simulink model "DIL_2025a"  (R2025a)
settings: Solver=VariableStepAuto  StartTime=0.0  StopTime=inf  FixedStep=.01  RelTol=1e-2
values from neighbouring files (symbols this model uses):
  s0 = load("s0.mat").s1(1:22)    [DIL_matlab.m]    (also in setup.m = load("s0.mat").s1(1:18)')
libraries: sl3dlib x1, sim3dlib x1, sim3dautolib x1
settings Model: Creator=Inver  LastModifiedBy=TAK
settings SolverCC: SolverJacobianMethodControl=FullAnalytical  DaesscMode=Robust  ZeroCrossAlgorithm=Adaptive
settings RTWCC: GPUComputeCapability=3.5

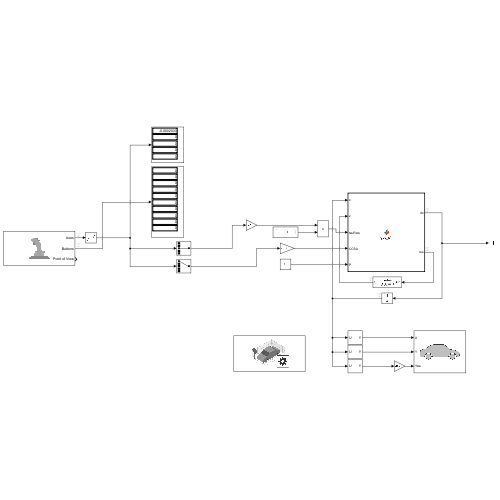
[thumbnail: Simulink's stored preview of the top-level diagram]
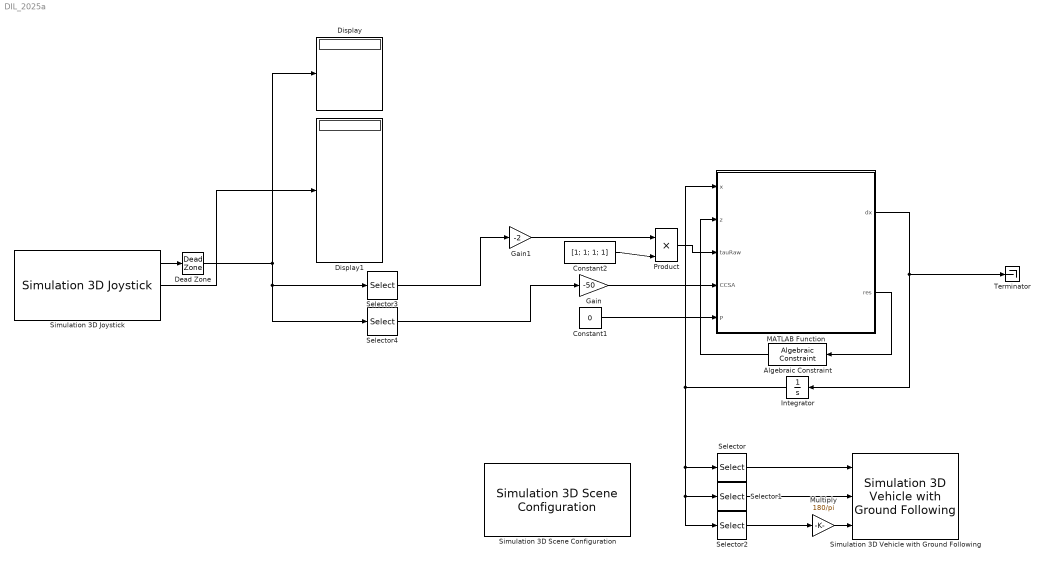
== system DIL_2025a ==
  Algebraic Constraint : AlgebraicConstraint  Tolerance=1e-6  InitialGuess=zeros(4, 1)
  Constant1 : Constant  Value=0
  Constant2 : Constant  Value=[1; 1; 1; 1]
  Dead Zone : DeadZone  LowerValue=-.02  UpperValue=.02
  Display : Display
  Display1 : Display
  Gain : Gain  Gain=-50
  Gain1 : Gain  Gain=-2
  Integrator : Integrator  InitialCondition=s0(1:18)
  MATLAB Function : MATLAB Function  TreatAsAtomicUnit=on
  Multiply : Gain  Gain=180/pi
  Product : Product
  Selector : Selector  InputPortWidth=18  IndexOptions=Index vector (dialog)  Indices=2  OutputSizes=1
  Selector1 : Selector  InputPortWidth=18  IndexOptions=Index vector (dialog)  Indices=4  OutputSizes=1
  Selector2 : Selector  InputPortWidth=18  IndexOptions=Index vector (dialog)  Indices=12  OutputSizes=1
  Selector3 : Selector  InputPortWidth=5  IndexOptions=Index vector (dialog)  Indices=3  OutputSizes=1
  Selector4 : Selector  InputPortWidth=5  IndexOptions=Index vector (dialog)  Indices=1  OutputSizes=1
  Simulation 3D Joystick : sl3dlib/Simulation 3D/Hardware Interface/Simulation 3D Joystick  joyid=1  adjustports=on  forcefeed=off
  Simulation 3D Scene Configuration : sim3dlib/Simulation 3D Scene Configuration  Priority=0  ProjectFormat=Default Scenes  SceneDesc=Double lane change  ProjectName=C:\Program Files\MATLAB\R2025a\toolbox\shared\sim3d_projects\automotive_project_windows\UE\WindowsNoEditor\VehicleSimulation.exe  ScenePath=/Game/Maps/HwStrght  EnableOpenDRIVE=off  vehTagList={'Custom';'Scene Origin';'SimulinkVehicle1'}  vehTag=SimulinkVehicle1  AttachedCameraRelativeTranslation=[0 0 10]  FreeCameraDefaultInitialTranslation=[-6, 0, 2]  AttachedCameraRelativeRotation=[0 -90 0]  FreeCameraDefaultInitialRotation=[0, -15, 0]  ViewpointName=Custom  FreeCameraInitialTranslation=[1182 -347 -230.5]  ViewpointTranslation=[0 0 0]  FreeCameraInitialRotation=[0 0 0]  ViewpointRotation=[0 0 0]  OpVisEn=off  Ts=.02  EnableWindow=on  EnableRemoteAccess=off  EnableWeather=off  SunAzimuth=90  SunAltitude=40.0  EnableGeospatialSun=off  Latitude=0  Longitude=0  Date=2023-01-01  Time=10:30:00  GeoTimeZone=-5.0  SunDaylightSaving=off  wind=1  clouds=10  EnableVolumetricClouds=off  CloudCoverage=0  CloudAltitude=6  fog=0  rain=0  RaindropsEffect=off  SnowDensity=0  EnableGeospatial=off  TilesetSource=Earth terrain  UseTrueOrigin=off  OriginHeight=200  OriginLatitude=40.744652  OriginLongitude=-73.988864  MapStyle=Aerial  AdditionalAssetIDs=[]  UseAdvancedSunSky=off  SolarTime=11  TimeZone=-5  Day=21  Month=9  Year=2022  UseDaylightSavingTime=on  DSTStartDay=10  DSTStartMonth=3  DSTEndDay=3  DSTEndMonth=11  DSTSwitchHour=2  sensorTag=MainCamera1  sensorId=1  sensorName=MainCamera1  mountLoc=Origin  offsetFlag=off  tmountOffset=[0, 0, 0]  rmountOffset=[0, 0, 0]  HorizontalResolution=1280  VerticalResolution=720  HorizontalFOV=60  mountPoint=[0 0 0]  mountOrientation=[0 0 0]  aMode=5  ID=1  GeoTrigger=Inactive  ViewNameList={'Custom'}  ViewTranslationList={'[1182 -347 -230.5]'}  ViewRotationList={'[0 0 0]'}
      settings: LibrarySourceBlock=sl3dlib/Simulation 3D/Environment/Simulation 3D Scene Configuration
  Simulation 3D Vehicle with Ground Following : sim3dautolib/Simulation 3D Vehicle with Ground Following  Priority=-1  PassVehMesh=Muscle car  MeshPath=/MathWorksAutomotiveContent/Vehicles/Muscle/Meshes/SK_MuscleCar.SK_MuscleCar  TrackWidth=1.9  WheelBase=3  WheelRadius=0.35  VehColor=Red  CoordinateSystem=ISO8855  InitialPos=[0, 0, 0]  InitialRot=[0, 0, 0]  ActorName=SimulinkVehicle1  SampleTime=-1  ActorType=SimulinkVehicle  ID=1  aMode=3  ActorTag=SimulinkVehicle1  CoordinateScheme=0  VehLightsControl=off  HeadlightColor=[ 1, 1, 1 ]  HighBeamIntensity=100000  LowBeamIntensity=60000  HighBeamConeAngle=70  LowBeamConeAngle=70  LeftHeadlightOrientation=[ 0, 0 ]  RightHeadlightOrientation=[ 0, 0 ]  BrakelightIntensity=500  ReverselightIntensity=500  SignallightIntensity=500  SignallightPeriod=1  SignalPulseWidth=50  TransformOutportEnabled=off
      settings: LibrarySourceBlock=drivingsim3d/Simulation 3D Vehicle with Ground Following
  Terminator : Terminator
  wires:
  MATLAB Function/1(dx) -> Integrator/1, Terminator/1
  Integrator/1 -> Selector/1, Selector1/1, Selector2/1, MATLAB Function/1(x)
  Gain/1 -> MATLAB Function/4(CCSA)
  Constant1/1 -> MATLAB Function/5(P)
  Constant2/1 -> Product/2
  MATLAB Function/2(res) -> Algebraic Constraint/1
  Algebraic Constraint/1 -> MATLAB Function/2(z)
  Selector/1 -> Simulation 3D Vehicle with Ground Following/1
  Selector1/1 -> Simulation 3D Vehicle with Ground Following/2
  Selector2/1 -> Multiply/1
  Multiply/1 -> Simulation 3D Vehicle with Ground Following/3
  Simulation 3D Joystick/1 -> Dead Zone/1
  Simulation 3D Joystick/2 -> Display1/1
  Product/1 -> MATLAB Function/3(tauRaw)
  Selector3/1 -> Gain1/1
  Selector4/1 -> Gain/1
  Dead Zone/1 -> Selector4/1, Selector3/1, Display/1
  Gain1/1 -> Product/1

== matlab function DIL_2025a/MATLAB Function ==
  data: x input; z input; dx output; tauRaw input; CCSA input; P input; varCAR parameter; res output
function [dx, res] = get_s1(x, z, tauRaw, CCSA, P, varCAR)
    s = [x; z];

    [xS, yS, zS, dxS, dyS, dzS, xT, yT, zT] = vehicle_suspension(s, varCAR);
    [SA, w] = vehicle_slip(s, CCSA, xT, yT, varCAR);
    [sum_Fxa, sum_Fya, sum_Fza, sum_Mx, sum_My, sum_Mz, res_torque] = vehicle_forces(s, CCSA, P, w, SA, xT, yT, zS, dzS, tauRaw, varCAR);
    derivatives = vehicle_dynamics(s, sum_Fxa, sum_Fya, sum_Fza, sum_Mx, sum_My, sum_Mz, res_torque, varCAR);
    [dVb, dAs, dT] = vehicle_powertrain(s, tauRaw, w, varCAR);

    dx = [derivatives; dVb; dAs; dT];
    res = res_torque;

    ds = [dx; res];

    if sum(isnan(ds)) || sum(isinf(ds))
        stop = 1;
    end
end
